simulink model "ProjectPenpulum_Simulink"  (R2023a)
settings: Solver=VariableStepAuto  StartTime=0.0  StopTime=10  MaxStep=0.01  RelTol=1e-3
model workspace (MAT data in the model file):
  Kf = 5
  g = 9.8
  l = 0.5
settings Model: NumberOfSteps=10  SnapshotBufferSize=50  PacingRate=2  Creator=hyyxl  LastModifiedBy=hyyxl

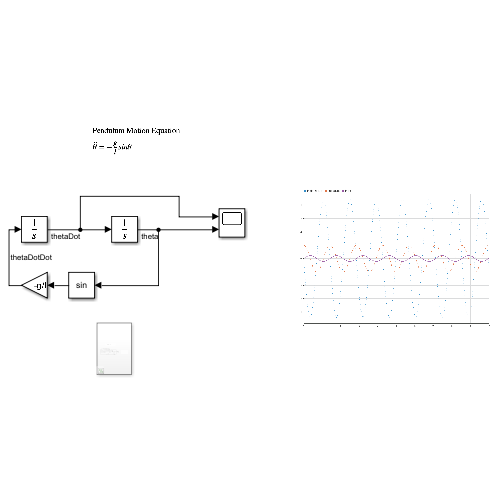
[thumbnail: Simulink's stored preview of the top-level diagram]
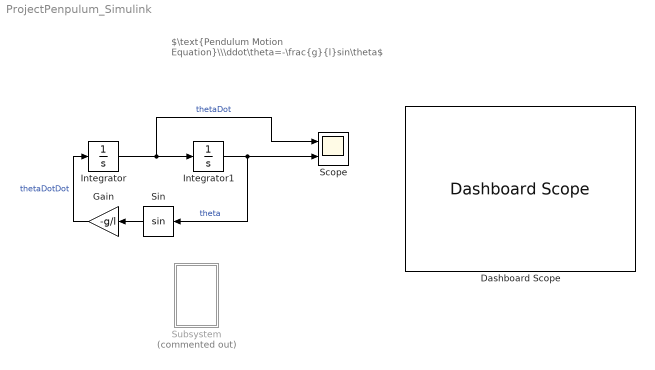
== system ProjectPenpulum_Simulink ==
  note: $\text{Pendulum Motion Equation}\\\ddot\theta=-\frac{g}{l}sin\theta$
  Dashboard Scope : DashboardScope
  Gain : Gain  Gain=-g/l
  Integrator : Integrator  InitialCondition=1
  Integrator1 : Integrator
  Scope : Scope  NumInputPorts=2
  Sin : Trigonometry
  Subsystem : Subsystem  Commented=on
  wires:
  Integrator/1 -> Scope/1, Integrator1/1  "thetaDot"
  Integrator1/1 -> Sin/1, Scope/2  "theta"
  Sin/1 -> Gain/1
  Gain/1 -> Integrator/1  "thetaDotDot"

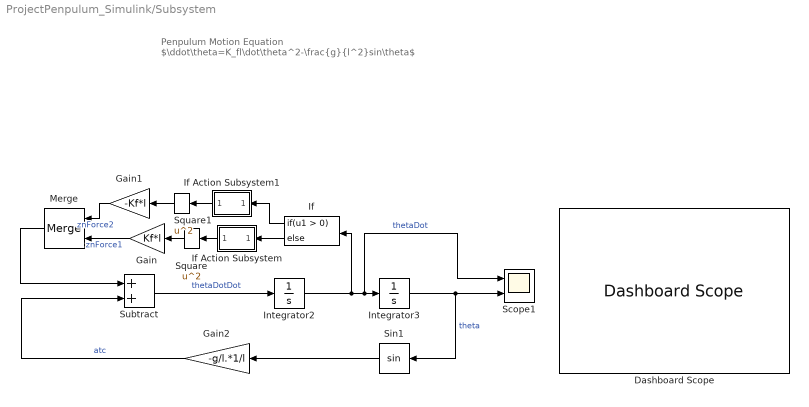
== system ProjectPenpulum_Simulink/Subsystem ==
  note: Penpulum Motion Equation
      |
      | $\ddot\theta=K_fl\dot\theta^2-\frac{g}{l^2}sin\theta$
  Dashboard Scope : DashboardScope
  Gain : Gain  Gain=Kf*l
  Gain1 : Gain  Gain=-Kf*l
  Gain2 : Gain  Gain=-g/l.*1/l
  If : If
  If Action Subsystem : Subsystem  TreatAsAtomicUnit=on
  If Action Subsystem1 : Subsystem  TreatAsAtomicUnit=on
  Integrator2 : Integrator  InitialCondition=0.8
  Integrator3 : Integrator
  Merge : Merge
  Scope1 : Scope  NumInputPorts=2
  Sin1 : Trigonometry
  Square : Math  Operator=square
  Square1 : Math  Operator=square
  Subtract : Sum
  wires:
  Sin1/1 -> Gain2/1
  Integrator3/1 -> Scope1/2, Sin1/1  "theta"
  Integrator2/1 -> If/1, Integrator3/1, Scope1/1  "thetaDot"
  Subtract/1 -> Integrator2/1  "thetaDotDot"
  If/2 -> If Action Subsystem/1(In1)
  Square/1 -> Gain/1
  Square1/1 -> Gain1/1
  If/1 -> If Action Subsystem1/1(In1)
  Gain2/1 -> Subtract/2  "atc"
  If Action Subsystem/1(Out1) -> Square/1
  If Action Subsystem1/1(Out1) -> Square1/1
  Gain1/1 -> Merge/1  "znForce2"
  Gain/1 -> Merge/2  "znForce1"
  Merge/1 -> Subtract/1

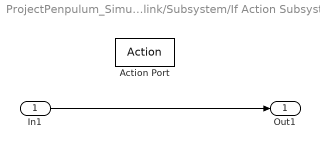
== system ProjectPenpulum_Simulink/Subsystem/If Action Subsystem ==
  In1 : Inport
  Action Port : ActionPort
  Out1 : Outport
  wires:
  In1/1 -> Out1/1

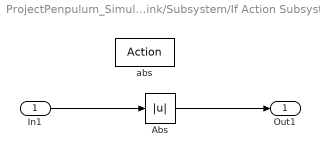
== system ProjectPenpulum_Simulink/Subsystem/If Action Subsystem1 ==
  In1 : Inport
  abs : ActionPort
  Abs : Abs  SaturateOnIntegerOverflow=off
  Out1 : Outport
  wires:
  In1/1 -> Abs/1
  Abs/1 -> Out1/1
